simulink model "UNIFIER1"  (R2023b)
settings: Solver=ode1  StartTime=0.0  StopTime=t_sim  FixedStep=1/500  RelTol=1e-3
values from neighbouring files (symbols this model uses):
  b = 20.11467    [UNIFIERLanding_20240613_190735.mat]    (also in UNIFIER_LOAD.m; UNIFIER_LOADsim.m; UNIFIER_trim_out_20240612_032607.mat)
  c = 1.43676    [UNIFIERLanding_20240613_190735.mat]    (also in UNIFIER_LOAD.m; UNIFIER_LOADsim.m; UNIFIER_trim_out_20240612_032607.mat)
  DEP_INTEG_IC = 117.49388    [UNIFIER_LOAD.m]    (also in UNIFIER_LOADsim.m; UNIFIER_trim_out_20240612_032607.mat)
  dp_DEP =     [UNIFIERLanding_20240613_190735.mat]    (also in UNIFIER_trim_out_20240612_032607.mat)
  dp_FUSE_FIN =     [UNIFIER_trim_out_20240612_032607.mat]
  dp_HTU =     [UNIFIERLanding_20240613_190735.mat]    (also in UNIFIER_trim_out_20240612_032607.mat)
  dp_VTAIL =     [UNIFIER_trim_out_20240612_032607.mat]
  dp_VTAIL_INDUCED =     [UNIFIER_trim_out_20240612_032607.mat]
  dp_WING_root =     [UNIFIER_trim_out_20240612_032607.mat]
  dp_WING_tip =     [UNIFIER_trim_out_20240612_032607.mat]
  dumax = [1.0471975512 1.0471975512 1.0471975512 0.174532925199 2 2 2]    [UNIFIERLanding_20240613_190735.mat]
  Euler0 = xstar(7:9)'    [UNIFIER_6DOFsim_init.m]    (also in UNIFIER_LOAD.m = [0, 0, 0]; UNIFIER_LOADsim.m; UNIFIER_trim_out_20240612_032607.mat = [3.43106170069e-06 0.0515008506278 -2.79252663434])
  ground_alt = 0    [UNIFIER_LOAD.m]    (also in UNIFIER_LOADsim.m; UNIFIER_trim_out_20240612_032607.mat)
  m = 7057    [UNIFIERLanding_20240613_190735.mat]    (also in UNIFIER_LOAD.m; UNIFIER_LOADsim.m; UNIFIER_trim_out_20240612_032607.mat)
  omegab0 = xstar(10:12)'    [UNIFIER_6DOFsim_init.m]    (also in UNIFIER_LOAD.m = [0,0,0]; UNIFIER_LOADsim.m; UNIFIER_trim_out_20240612_032607.mat = [0 0 0])
  S = 29.98388    [UNIFIERLanding_20240613_190735.mat]    (also in UNIFIER_LOAD.m; UNIFIER_LOADsim.m; UNIFIER_trim_out_20240612_032607.mat)
  sensor_delay_steps = 5    [UNIFIER_LOAD.m]    (also in UNIFIER_LOADsim.m; UNIFIER_trim_out_20240612_032607.mat)
  solution =     [UNIFIERLanding_20240613_190735.mat]
  u1_0 = [ustar(1), -1*ustar(1), ustar(3)-ustar(2), ustar(3)+ustar(2), ustar(4), ustar(4)]    [UNIFIER_6DOFsim_init.m]    (also in UNIFIER_LOAD.m = [2.1112539e-05, -2.1112539e-05, -0.085004635, -0.084972650, ; UNIFIER_LOADsim.m = [2.1112539e-05, -2.1112539e-05, -0.085004635, -0.084972650, ; UNIFIER_trim_out_20240612_032607.mat = [2.1112539e-05 -2.1112539e-05 -0.085004635 -0.08497265 0.197)
  u2_0 = ones(1,12) .* ustar(5)    [UNIFIER_6DOFsim_init.m]    (also in UNIFIER_LOAD.m = ones(1,12) .* 0.4252; UNIFIER_LOADsim.m = ones(1,12) .* 0.4252; UNIFIER_trim_out_20240612_032607.mat = [0.4252 0.4252 0.4252 0.4252 0.4252 0.4252 0.4252 0.4252 0.4)
  u3_0 = ustar(7)    [UNIFIER_6DOFsim_init.m]    (also in UNIFIER_LOAD.m = 0.089689; UNIFIER_LOADsim.m = 0.089689; UNIFIER_trim_out_20240612_032607.mat = 0.089689)
  u4_0 = 0    [UNIFIER_6DOFsim_init.m]    (also in UNIFIER_LOAD.m; UNIFIER_LOADsim.m; UNIFIER_trim_out_20240612_032607.mat)
  u_trim = ustar    [UNIFIER_6DOFsim_init.m]    (also in UNIFIER_LOAD.m = [0.0; UNIFIER_LOADsim.m)
  umax = [0.436332312999 0.523598775598 0.523598775598 0.436332312999 1 1 1]    [UNIFIERLanding_20240613_190735.mat]    (also in UNIFIER_trim_out_20240612_032607.mat)
  umin = [-0.436332312999 -0.523598775598 -0.523598775598 0 0 -1 -0.5]    [UNIFIERLanding_20240613_190735.mat]    (also in UNIFIER_trim_out_20240612_032607.mat)
  Va = [72.7399985115 72.2978466179 70.3592089076 68.5755686022 67.5674222915 66.8967003826 65.8958642605 64.4243196248 62.667507398 61.0171213882 59.8601734245 59.2796795419 ... (250 elements, 250x1)]    [UNIFIERLanding_20240613_190735.mat]
  Vb0 = xstar(4:6)'    [UNIFIER_6DOFsim_init.m]    (also in UNIFIER_LOAD.m = [72.731047032614440, 0, 1.142307104518741]; UNIFIER_LOADsim.m; UNIFIER_trim_out_20240612_032607.mat = [52.6789583502 0 2.71559652634])
  vtail_dist_to_wing = 7.8070    (= 7.807)    [UNIFIER_LOAD.m]    (also in UNIFIER_LOADsim.m; UNIFIER_trim_out_20240612_032607.mat)
  vtail_nodes = [dp_VTAIL.Xs_LE;     dp_VTAIL.Ys_LE;     dp_VTAIL.Zs_LE]    [UNIFIER_LOAD.m]    (also in UNIFIER_LOADsim.m; UNIFIER_trim_out_20240612_032607.mat = [-16.4894695282 -2.83441376686 -2.73765826225 -16.1370849609)
  wing_nodes = [fliplr(dp_WING_tip.LE_Xs),fliplr(dp_WING_root.LE_Xs),dp_WING_root.LE_Xs,dp_WING_tip.LE_Xs;     fliplr(-dp_WING_tip.LE_Ys),fliplr(-dp_WING_root.LE_Ys),dp_WING_root.LE_Ys,dp_WING_tip.LE_Ys;     fliplr(dp_WING_tip.LE_Zs),fliplr(dp_WING_root.LE_Zs),dp_WING_root.LE_Zs,dp_WING_tip.LE_Zs]    [UNIFIER_LOAD.m]    (also in UNIFIER_LOADsim.m; UNIFIER_trim_out_20240612_032607.mat = [-7.70795631409 -9.67500019073 -0.98178178072 -7.66801691055)
  Xe0 = xstar(1:3)'    [UNIFIER_6DOFsim_init.m]    (also in UNIFIER_LOAD.m = [0,0,-1219]; UNIFIER_LOADsim.m; UNIFIER_trim_out_20240612_032607.mat = [0 0 -1100])
  xyz_cg = [-8.09 0 -0.2]    [UNIFIERLanding_20240613_190735.mat]    (also in UNIFIER_LOAD.m = [-8.09,0,-0.2]; UNIFIER_LOADsim.m = [-8.09,0,-0.2]; UNIFIER_trim_out_20240612_032607.mat)
  xyz_DEP = [-6.9629998 -10.05 -0.90899998 -6.921 -8.4499998 -0.792 -6.8660002 -6.8499999 -0.82300001 -6.8099999 -5.25 -0.85000002 ... (36 elements, 3x12)]    [UNIFIERLanding_20240613_190735.mat]    (also in UNIFIER_LOAD.m = [ -6.9629998	-6.9210000	-6.8660002	-6.8099999	-6.7540002	-6.; UNIFIER_LOADsim.m = [ -6.9629998	-6.9210000	-6.8660002	-6.8099999	-6.7540002	-6.; UNIFIER_trim_out_20240612_032607.mat)
undefined symbols (not defined in the file or in its folder): Earth, F, MIL, WGS84
libraries: simulink_extras x22, aerolibactuator x16, dspnetwork x15, sharedutil x14, sharedtransform x7, aerolibtransform2 x5, slpidlib x5, simulink x5, aerolibwind2 x4, matrix_library x1, shared6dof x1, aerolibatmos2 x1
(part 1 of 5)
settings Model: PauseTimes=1.5  Creator=johannes  LastModifiedBy=Reggie Johanes
settings DebuggingCC: ParameterPrecisionLossMsg=none  UnconnectedInputMsg=warning  UnconnectedOutputMsg=warning  UnconnectedLineMsg=warning  UnitsInconsistencyMsg=none  AllowAutomaticUnitConversions=off
settings ModelReferenceCC: EnableRefExpFcnMdlSchedulingChecks=on
settings RTWCC: DLArmComputeVersion=19.05

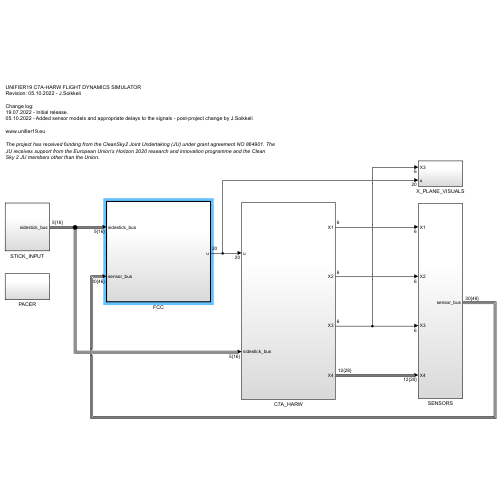
[thumbnail: Simulink's stored preview of the top-level diagram]
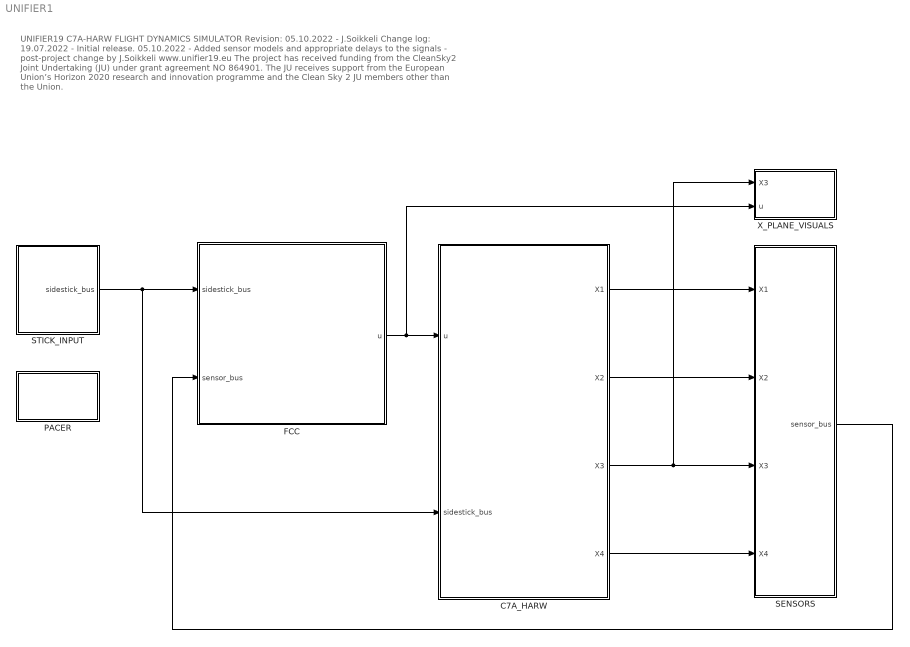
== system UNIFIER1 ==
  note: UNIFIER19 C7A-HARW FLIGHT DYNAMICS SIMULATOR
      | Revision: 05.10.2022 - J.Soikkeli
      |
      | Change log:
      | 19.07.2022 - Initial release.
      | 05.10.2022 - Added sensor models and appropriate delays to the signals - post-project change by J.Soikkeli
      |
      | www.unifier19.eu
      |
      | The project has received funding from the CleanSky2 Joint Undertaking (JU) under grant agreement NO 864901. The JU receives support from the European Union’s Horizon 2020 research and innovation programme and the Clean Sky 2 JU members other than the Union.
  C7A_HARW : Subsystem
  FCC : Subsystem  TreatAsAtomicUnit=on
  PACER : Subsystem
  SENSORS : Subsystem
  STICK_INPUT : Subsystem
  X_PLANE_VISUALS : Subsystem
  wires:
  C7A_HARW/3(X3) -> SENSORS/3(X3), X_PLANE_VISUALS/1(X3)
  FCC/1(u) -> X_PLANE_VISUALS/2(u), C7A_HARW/1(u)
  C7A_HARW/1(X1) -> SENSORS/1(X1)
  C7A_HARW/2(X2) -> SENSORS/2(X2)
  C7A_HARW/4(X4) -> SENSORS/4(X4)
  SENSORS/1(sensor_bus) -> FCC/2(sensor_bus)
  STICK_INPUT/1(sidestick_bus) -> C7A_HARW/2(sidestick_bus), FCC/1(sidestick_bus)

== system UNIFIER1/C7A_HARW ==
  u : Inport
  sidestick_bus : Inport  Port=2
  Actuator processing and transport delay 10 ms : Delay  DelayLength=5  InitialCondition=repmat([u1_0,u2_0,u3_0,u4_0]',1,5)
  Aero : Subsystem
  Bus Selector : BusSelector  OutputSignals=V_rw_tas,omega_rw,V_rw_mag_tas,beta,alpha,rho
  Cast{1,6..12} (8 alike) : DataTypeConversion  OutDataTypeStr=single  SaturateOnIntegerOverflow=off  RndMeth=Floor
  Demux : Demux  Outputs=[6,12,1,1]
  EOMandEnviroment1 : Subsystem
  FCC frame delay 10 ms (assumed 100Hz FCC) : Delay  DelayLength=5  InitialCondition=repmat([u1_0,u2_0,u3_0,u4_0]',1,5)
  Scopes : Subsystem
  Subsystems : Subsystem
  Sum : Sum  Inputs=|++
  Sum1 : Sum  Inputs=|++
  X1 : Outport
  X2 : Outport  Port=2
  X3 : Outport  Port=3
  X4 : Outport  Port=4
  wires:
  Aero/2(M) -> Sum1/1
  Bus Selector/1 -> Cast7/1  "<V_rw_tas>"
  Bus Selector/6 -> Cast8/1  "<rho>"
  Bus Selector/2 -> Cast9/1  "<omega_rw>"
  Cast6/1 -> Aero/7(DEP_J)
  Subsystems/1(DEP_J) -> Cast6/1
  Subsystems/3(F) -> Sum/2
  Aero/1(F) -> Sum/1
  Sum/1 -> EOMandEnviroment1/1(F)
  Sum1/1 -> EOMandEnviroment1/2(M)
  Subsystems/4(M) -> Sum1/2
  Bus Selector/3 -> Cast10/1  "<V_rw_mag_tas>"
  Bus Selector/4 -> Cast11/1  "<beta>"
  Bus Selector/5 -> Cast12/1  "<alpha>"
  Cast7/1 -> Aero/1(V_rw_tas)
  Cast8/1 -> Aero/6(rho)
  Cast9/1 -> Aero/2(omega_rw)
  Cast10/1 -> Aero/3(V_rw_mag_tas)
  Cast11/1 -> Aero/4(beta)
  Cast12/1 -> Aero/5(alpha)
  Cast1/1 -> Aero/8(u1 (rad))
  Subsystems/2(u1_out (rad)) -> Cast1/1
  EOMandEnviroment1/1(X1) -> Scopes/1(X1), X1/1
  EOMandEnviroment1/4(X4) -> Scopes/4(X4), X4/1, Subsystems/1(X4), Bus Selector/1
  EOMandEnviroment1/2(X2) -> Subsystems/7(X2), X2/1, Scopes/2(X2)
  EOMandEnviroment1/3(X3) -> Subsystems/6(X3), X3/1, Scopes/3(X3)
  Demux/4 -> Aero/9(u4 (gear))
  sidestick_bus/1 -> Subsystems/5(sidestick_bus)
  Demux/3 -> Subsystems/4(u3 (actf))
  Demux/2 -> Subsystems/3(u2 (actf))
  Demux/1 -> Subsystems/2(u1_in (rad))
  u/1 -> FCC frame delay 10 ms (assumed 100Hz FCC)/1
  FCC frame delay 10 ms (assumed 100Hz FCC)/1 -> Actuator processing and transport delay 10 ms/1
  Actuator processing and transport delay 10 ms/1 -> Demux/1

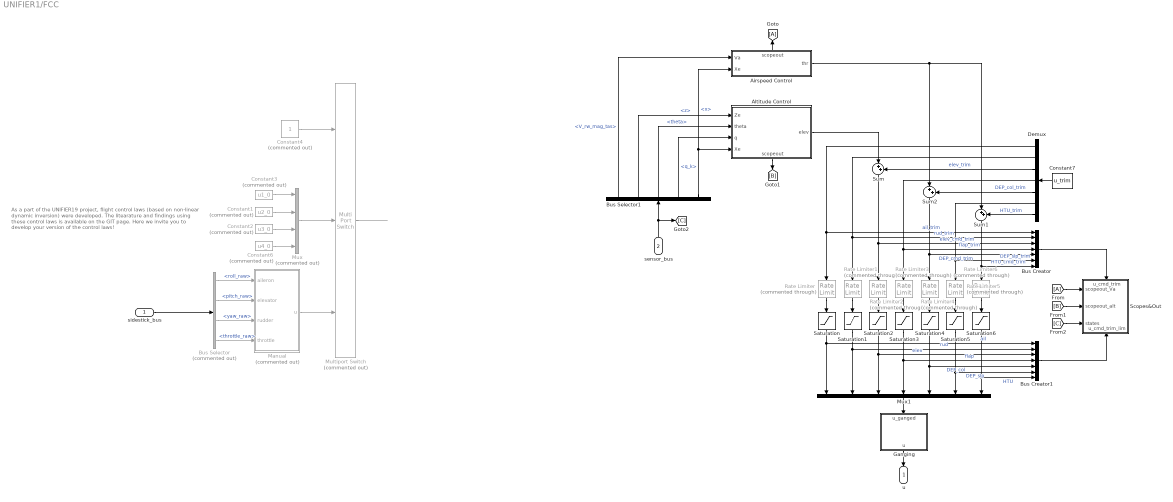
== system UNIFIER1/FCC ==
  note: As a part of the UNIFIER19 project, flight control laws (based on non-linear dynamic inversion) were developed. The litearature and findings using these control laws is available on the GIT page.
      |
      | Here we invite you to develop your version of the control laws!
  sidestick_bus : Inport
  sensor_bus : Inport  Port=2
  Airspeed Control : Subsystem
      settings: PortSchema="{\"entries\":[{\"content\":{\"sides\":[{\"content\":{\"connectorIds\":[\"In1\",\"In2\"]},\"type\":\"ConnectorPlacement.EquallySpacedRectSide\",\"uuid\":\"a3fb04a8-89c2-4134-89d4-6d6a43062b9b\"},{\"content\":{\"connectorIds\":[\"Out1\"],\"side\":\"RIGHT\"},\"type\":\"ConnectorPlacement.EquallySpacedRectSide\",\"uuid\":\"0d35a5ec-1bbb-45b5-ad25-2bc644cb46ec\"},{\"content\":{\"connectorIds\":[\"Out2\"],\"side\":\"TOP\"},\"type\":\"ConnectorPlacement.EquallySpacedRectSide\",\"uuid\":\"07800402-c5fd-46cf-bb6b-6507cb62190b\"}]},\"type\":\"ConnectorPlacement.EquallySpacedConnector\",\"uuid\":\"0f781fd0-6236-48b8-b612-1777b9bca292\"}],\"packageUris\":[\"http://schema.mathworks.com/mf0/Connector/R2020b\"],\"version\":\"1.0\"}"
  Altitude Control : Subsystem
      settings: PortSchema="{\"entries\":[{\"content\":{\"sides\":[{\"content\":{\"connectorIds\":[\"In1\",\"In2\",\"In3\",\"In4\"]},\"type\":\"ConnectorPlacement.EquallySpacedRectSide\",\"uuid\":\"d6eebd62-3574-4a6b-be51-6258a51c0c28\"},{\"content\":{\"connectorIds\":[\"Out1\"],\"side\":\"RIGHT\"},\"type\":\"ConnectorPlacement.EquallySpacedRectSide\",\"uuid\":\"54870a02-b95d-471b-a2c8-ee83b599c45e\"},{\"content\":{\"side\":\"TOP\"},\"type\":\"ConnectorPlacement.EquallySpacedRectSide\",\"uuid\":\"efdc830e-c8bf-412c-9d86-dbb1e6c1c86b\"},{\"content\":{\"connectorIds\":[\"Out2\"],\"side\":\"BOTTOM\"},\"type\":\"ConnectorPlacement.EquallySpacedRectSide\",\"uuid\":\"beb3ac17-a4c7-4320-a029-baa0478db22b\"}]},\"type\":\"ConnectorPlacement.EquallySpacedConnector\",\"uuid\":\"0f69f6a5-bc47-4551-ad8e-935190b4abb2\"}],\"packageUris\":[\"http://schema.mathworks.com/mf0/Connector/R2020b\"],\"version\":\"1.0\"}"
  Bus Creator : BusCreator  Inputs=7
  Bus Creator1 : BusCreator  Inputs=7
  Bus Selector : BusSelector  Commented=on  OutputSignals=roll_raw,pitch_raw,yaw_raw,throttle_raw
  Bus Selector1 : BusSelector  OutputSignals=V_rw_mag_tas,z,theta,q_k,x
  Constant1 : Constant  Commented=on  Value=u2_0
  Constant2 : Constant  Commented=on  Value=u3_0
  Constant3 : Constant  Commented=on  Value=u1_0
  Constant4 : Constant  Commented=on  SampleTime=-1
  Constant6 : Constant  Commented=on  Value=u4_0
  Constant7 : Constant  Value=u_trim
  Demux : Demux  Outputs=7
  From : From
  Ganging : Subsystem
  Goto : Goto
  Manual : Subsystem  Commented=on
  Multiport Switch : MultiPortSwitch  Commented=on  Inputs=2  SaturateOnIntegerOverflow=off  InputSameDT=off
  Mux : Mux  Commented=on
  Mux1 : Mux  Inputs=7
  Rate Limiter : RateLimiter  Commented=through  RisingSlewLimit=dumax(1)  FallingSlewLimit=-dumax(1)  SampleTimeMode=inherited
  Rate Limiter1 : RateLimiter  Commented=through  RisingSlewLimit=dumax(2)  FallingSlewLimit=-dumax(2)  SampleTimeMode=inherited
  Rate Limiter2 : RateLimiter  Commented=through  RisingSlewLimit=dumax(3)  FallingSlewLimit=-dumax(3)  SampleTimeMode=inherited
  Rate Limiter3 : RateLimiter  Commented=through  RisingSlewLimit=dumax(4)  FallingSlewLimit=-dumax(4)  SampleTimeMode=inherited
  Rate Limiter4 : RateLimiter  Commented=through  RisingSlewLimit=dumax(5)  FallingSlewLimit=-dumax(5)  SampleTimeMode=inherited
  Rate Limiter5 : RateLimiter  Commented=through  RisingSlewLimit=dumax(6)  FallingSlewLimit=-dumax(6)  SampleTimeMode=inherited
  Rate Limiter6 : RateLimiter  Commented=through  RisingSlewLimit=dumax(7)  FallingSlewLimit=-dumax(7)  SampleTimeMode=inherited
  Saturation : Saturate  UpperLimit=umax(1)  LowerLimit=umin(1)
  Saturation1 : Saturate  UpperLimit=umax(2)  LowerLimit=umin(2)
  Saturation2 : Saturate  UpperLimit=umax(3)  LowerLimit=umin(3)
  Saturation3 : Saturate  UpperLimit=umax(4)  LowerLimit=umin(4)
  Saturation4 : Saturate  UpperLimit=umax(5)  LowerLimit=umin(5)
  Saturation5 : Saturate  UpperLimit=umax(6)  LowerLimit=umin(6)
  Saturation6 : Saturate  UpperLimit=umax(7)  LowerLimit=umin(7)
  Scopes&Out : Subsystem
      settings: PortSchema="{\"entries\":[{\"content\":{\"sides\":[{\"content\":{\"connectorIds\":[\"In1\",\"In2\",\"In3\"]},\"type\":\"ConnectorPlacement.EquallySpacedRectSide\",\"uuid\":\"9c320b89-1cdf-46a8-9001-4899d9265a08\"},{\"content\":{\"side\":\"RIGHT\"},\"type\":\"ConnectorPlacement.EquallySpacedRectSide\",\"uuid\":\"9f59574f-7d1d-4902-b616-eb94195d59ee\"},{\"content\":{\"connectorIds\":[\"In4\"],\"side\":\"TOP\"},\"type\":\"ConnectorPlacement.EquallySpacedRectSide\",\"uuid\":\"0802dcde-7117-4a51-8755-c38da5aaf345\"},{\"content\":{\"connectorIds\":[\"In5\"],\"side\":\"BOTTOM\"},\"type\":\"ConnectorPlacement.EquallySpacedRectSide\",\"uuid\":\"322f023d-fcca-4329-b22d-247bcb46a2a3\"}]},\"type\":\"ConnectorPlacement.EquallySpacedConnector\",\"uuid\":\"183cf95f-4342-4e51-9921-cf7b583031df\"}],\"packageUris\":[\"http://schema.mathworks.com/mf0/Connector/R2020b\"],\"version\":\"1.0\"}"
  Sum : Sum  Inputs=|++
  Sum1 : Sum  Inputs=|++
  Sum2 : Sum  Inputs=|++
  u : Outport
  wires:
  Multiport Switch/1 -> ?
  Constant3/1 -> Mux/1
  Constant1/1 -> Mux/2
  Constant2/1 -> Mux/3
  Mux/1 -> Multiport Switch/2
  Bus Selector/1 -> Manual/1(aileron)  "<roll_raw>"
  Bus Selector/2 -> Manual/2(elevator)  "<pitch_raw>"
  Bus Selector/3 -> Manual/3(rudder)  "<yaw_raw>"
  Bus Selector/4 -> Manual/4(throttle)  "<throttle_raw>"
  Constant4/1 -> Multiport Switch/1
  Manual/1(u) -> Multiport Switch/3
  Constant6/1 -> Mux/4
  sidestick_bus/1 -> Bus Selector/1
  sensor_bus/1 -> Bus Selector1/1, [C]
  Ganging/1(u) -> u/1
  Bus Selector1/2 -> Altitude Control/1(Ze)  "<z>"
  Bus Selector1/3 -> Altitude Control/2(theta)  "<theta>"
  Bus Selector1/4 -> Altitude Control/3(q)  "<q_k>"
  Bus Selector1/1 -> Airspeed Control/1(Va)  "<V_rw_mag_tas>"
  Mux1/1 -> Ganging/1(u_ganged)
  Altitude Control/1(elev) -> Sum/1
  Airspeed Control/1(thr) -> Sum1/1, Sum2/1
  Saturation/1 -> Mux1/1, Bus Creator1/1  "ail"
  Saturation1/1 -> Mux1/2, Bus Creator1/2  "rud"
  Saturation2/1 -> Mux1/3, Bus Creator1/3  "elev"
  Saturation3/1 -> Mux1/4, Bus Creator1/4  "flap"
  Saturation4/1 -> Mux1/5, Bus Creator1/5  "DEP_col"
  Saturation5/1 -> Mux1/6, Bus Creator1/6  "DEP_slp"
  Saturation6/1 -> Mux1/7, Bus Creator1/7  "HTU"
  Constant7/1 -> Demux/1
  Demux/1 -> Bus Creator/1, Rate Limiter/1  "ail_trim"
  Demux/2 -> Bus Creator/2, Rate Limiter1/1  "rud_trim"
  Demux/3 -> Sum/2  "elev_trim"
  Demux/4 -> Bus Creator/4, Rate Limiter3/1  "flap_trim"
  Demux/5 -> Sum2/2  "DEP_col_trim"
  Demux/6 -> Bus Creator/6, Rate Limiter5/1  "DEP_slp_trim"
  Demux/7 -> Sum1/2  "HTU_trim"
  Bus Selector1/5 -> Altitude Control/4(Xe), Airspeed Control/2(Xe)  "<x>"
  Sum/1 -> Rate Limiter2/1, Bus Creator/3  "elev_cmd_trim"
  Sum1/1 -> Rate Limiter6/1, Bus Creator/7  "HTU_cmd_trim"
  Sum2/1 -> Rate Limiter4/1, Bus Creator/5  "DEP_cmd_trim"
  Rate Limiter/1 -> Saturation/1
  Rate Limiter1/1 -> Saturation1/1
  Rate Limiter2/1 -> Saturation2/1
  Rate Limiter3/1 -> Saturation3/1
  Rate Limiter4/1 -> Saturation4/1
  Rate Limiter5/1 -> Saturation5/1
  Rate Limiter6/1 -> Saturation6/1
  Altitude Control/2(scopeout) -> [B]
  Airspeed Control/2(scopeout) -> Goto/1
  From/1 -> Scopes&Out/1(scopeout_Va)
  [B] -> Scopes&Out/2(scopeout_alt)
  Bus Creator/1 -> Scopes&Out/4(u_cmd_trim)
  Bus Creator1/1 -> Scopes&Out/5(u_cmd_trim_lim)
  [C] -> Scopes&Out/3(states)

== system UNIFIER1/PACER ==
  note: Soft real time block and associated
      | s-function source codes:
      | - sfun_sleep.c
      | - sfun_getSystemClockTimeval.c
      | - sfun_output_to_console.c
      | are copyrighted
      | by Marc Compere
      | comperem@gmail.com
      | created : 28 May 2018
      | modified: 28 May 2018
  Constant1 : Constant  Value=0
  Constant2 : Constant
  Display : Display
  Manual Switch1 : ManualSwitch  CurrentSetting=0
  Mux : Mux  Inputs=3
  Output to Console : Subsystem  TreatAsAtomicUnit=on
  Subsystem : Subsystem
      settings: OpenFcn=h_fixed=0.001
      mask Display: fprintf('Double-Click to init\nstepsize variable, h_fixed')
  "pace error (s) " : Scope
  simulation time (s)1 : Clock
  soft real time subsystem : Subsystem  mask{t_sample=0.01}
      mask prompts: t_sample "Sleep function interval (s)"
  wires:
  soft real time subsystem/2(pace error (s)) -> "pace error (s) "/1, Display/1, Mux/3
  simulation time (s)1/1 -> Mux/1
  soft real time subsystem/1(t_elapsed_wall_clock (s)) -> Mux/2
  Constant1/1 -> Manual Switch1/2
  Mux/1 -> Output to Console/1(data to console)
  Constant2/1 -> Manual Switch1/1
  Manual Switch1/1 -> Output to Console/Enable

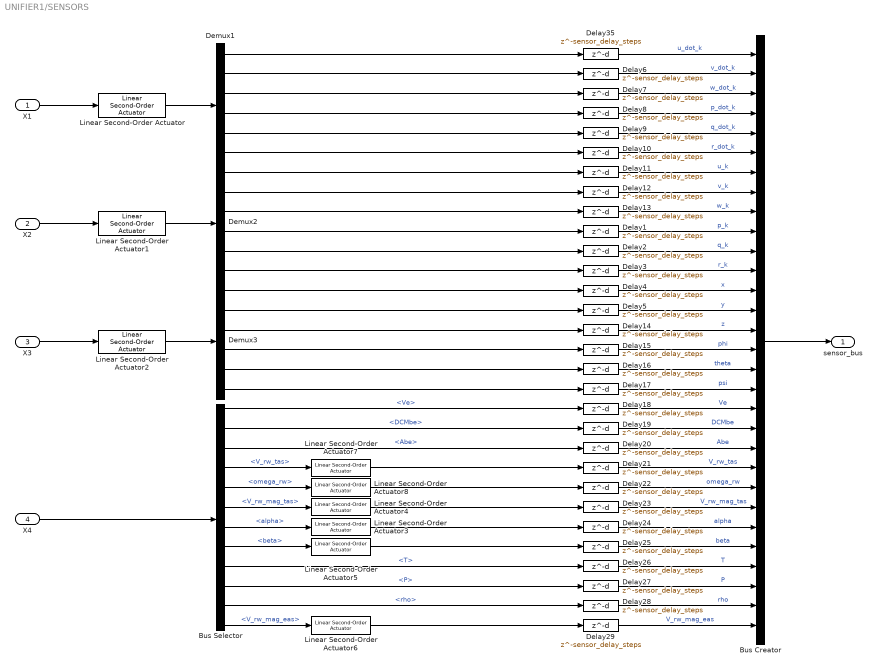
== system UNIFIER1/SENSORS ==
  X1 : Inport
  X2 : Inport  Port=2
  X3 : Inport  Port=3
  X4 : Inport  Port=4
  Bus Creator : BusCreator  Inputs=30
  Bus Selector : BusSelector  OutputSignals=Ve,DCMbe,Abe,V_rw_tas,omega_rw,V_rw_mag_tas,alpha,beta,T,P,rho,V_rw_mag_eas
  Delay{1..3,6..10,35} (9 alike) : Delay  DelayLength=sensor_delay_steps
  Delay11 : Delay  DelayLength=sensor_delay_steps  InitialCondition=Vb0(1)
  Delay12 : Delay  DelayLength=sensor_delay_steps  InitialCondition=Vb0(2)
  Delay13 : Delay  DelayLength=sensor_delay_steps  InitialCondition=Vb0(3)
  Delay14 : Delay  DelayLength=sensor_delay_steps  InitialCondition=Xe0(3)
  Delay15 : Delay  DelayLength=sensor_delay_steps  InitialCondition=Euler0(1)
  Delay16 : Delay  DelayLength=sensor_delay_steps  InitialCondition=Euler0(2)
  Delay17 : Delay  DelayLength=sensor_delay_steps  InitialCondition=Euler0(3)
  Delay18 : Delay  DelayLength=sensor_delay_steps  InitialCondition=repmat(Vb0',1,sensor_delay_steps)
  Delay19 : Delay  DelayLength=sensor_delay_steps  InitialCondition=0
  Delay20 : Delay  DelayLength=sensor_delay_steps  InitialCondition=0
  Delay21 : Delay  DelayLength=sensor_delay_steps  InitialCondition=repmat(Vb0',1,sensor_delay_steps)
  Delay22 : Delay  DelayLength=sensor_delay_steps  InitialCondition=0
  Delay23 : Delay  DelayLength=sensor_delay_steps  InitialCondition=sqrt(dot(Vb0,Vb0))
  Delay24 : Delay  DelayLength=sensor_delay_steps  InitialCondition=atan(Vb0(3)/Vb0(1))
  Delay25 : Delay  DelayLength=sensor_delay_steps  InitialCondition=asin(Vb0(2)/sqrt(dot(Vb0,Vb0)))
  Delay26 : Delay  DelayLength=sensor_delay_steps  InitialCondition=273
  Delay27 : Delay  DelayLength=sensor_delay_steps  InitialCondition=101325
  Delay28 : Delay  DelayLength=sensor_delay_steps  InitialCondition=1.225
  Delay29 : Delay  DelayLength=sensor_delay_steps  InitialCondition=sqrt(dot(Vb0,Vb0))
  Delay4 : Delay  DelayLength=sensor_delay_steps  InitialCondition=Xe0(1)
  Delay5 : Delay  DelayLength=sensor_delay_steps  InitialCondition=Xe0(2)
  Demux1 : Demux  Outputs=6
  Demux2 : Demux  Outputs=6
  Demux3 : Demux  Outputs=6
  Linear Second-Order Actuator : aerolibactuator/Linear Second-Order Actuator  wn_fin=30*2*pi  z_fin=1  fin_act_0=zeros(1,6)  fin_act_vel=0
  Linear Second-Order Actuator1 : aerolibactuator/Linear Second-Order Actuator  wn_fin=30*2*pi  z_fin=1  fin_act_0=[Vb0,omegab0]  fin_act_vel=0
  Linear Second-Order Actuator2 : aerolibactuator/Linear Second-Order Actuator  wn_fin=30*2*pi  z_fin=1  fin_act_0=[Xe0,Euler0]  fin_act_vel=0
  Linear Second-Order Actuator3 : aerolibactuator/Linear Second-Order Actuator  wn_fin=5*2*pi  z_fin=1  fin_act_0=atan(Vb0(3)/Vb0(1))  fin_act_vel=0
  Linear Second-Order Actuator4 : aerolibactuator/Linear Second-Order Actuator  wn_fin=5*2*pi  z_fin=1  fin_act_0=sqrt((Vb0(1)^2+Vb0(2)^2+Vb0(3)^2))  fin_act_vel=0
  Linear Second-Order Actuator5 : aerolibactuator/Linear Second-Order Actuator  wn_fin=5*2*pi  z_fin=1  fin_act_0=asin(Vb0(2)/sqrt((Vb0(1)^2+Vb0(2)^2+Vb0(3)^2)))  fin_act_vel=0
  Linear Second-Order Actuator6 : aerolibactuator/Linear Second-Order Actuator  wn_fin=5*2*pi  z_fin=1  fin_act_0=sqrt((Vb0(1)^2+Vb0(2)^2+Vb0(3)^2))  fin_act_vel=0
  Linear Second-Order Actuator7 : aerolibactuator/Linear Second-Order Actuator  wn_fin=5*2*pi  z_fin=1  fin_act_0=Vb0  fin_act_vel=0
  Linear Second-Order Actuator8 : aerolibactuator/Linear Second-Order Actuator  wn_fin=30*2*pi  z_fin=1  fin_act_0=omegab0  fin_act_vel=0
  sensor_bus : Outport
  wires:
  Demux1/1 -> Delay35/1
  Demux1/2 -> Delay6/1
  X4/1 -> Bus Selector/1
  Bus Selector/4 -> Linear Second-Order Actuator7/1  "<V_rw_tas>"
  Bus Selector/5 -> Linear Second-Order Actuator8/1  "<omega_rw>"
  Bus Selector/6 -> Linear Second-Order Actuator4/1  "<V_rw_mag_tas>"
  Bus Selector/7 -> Linear Second-Order Actuator3/1  "<alpha>"
  Bus Selector/8 -> Linear Second-Order Actuator5/1  "<beta>"
  Bus Selector/12 -> Linear Second-Order Actuator6/1  "<V_rw_mag_eas>"
  X1/1 -> Linear Second-Order Actuator/1
  X2/1 -> Linear Second-Order Actuator1/1
  X3/1 -> Linear Second-Order Actuator2/1
  Linear Second-Order Actuator/1 -> Demux1/1
  Linear Second-Order Actuator1/1 -> Demux2/1
  Linear Second-Order Actuator2/1 -> Demux3/1
  Bus Creator/1 -> sensor_bus/1
  Linear Second-Order Actuator6/1 -> Delay29/1
  Bus Selector/11 -> Delay28/1  "<rho>"
  Bus Selector/10 -> Delay27/1  "<P>"
  Bus Selector/9 -> Delay26/1  "<T>"
  Linear Second-Order Actuator5/1 -> Delay25/1
  Linear Second-Order Actuator3/1 -> Delay24/1
  Linear Second-Order Actuator4/1 -> Delay23/1
  Linear Second-Order Actuator8/1 -> Delay22/1
  Linear Second-Order Actuator7/1 -> Delay21/1
  Bus Selector/3 -> Delay20/1  "<Abe>"
  Bus Selector/2 -> Delay19/1  "<DCMbe>"
  Bus Selector/1 -> Delay18/1  "<Ve>"
  Demux3/6 -> Delay17/1
  Demux3/5 -> Delay16/1
  Demux3/4 -> Delay15/1
  Demux3/3 -> Delay14/1
  Demux3/2 -> Delay5/1
  Demux3/1 -> Delay4/1
  Demux2/6 -> Delay3/1
  Demux2/5 -> Delay2/1
  Demux2/4 -> Delay1/1
  Demux2/3 -> Delay13/1
  Demux2/2 -> Delay12/1
  Demux2/1 -> Delay11/1
  Demux1/6 -> Delay10/1
  Demux1/5 -> Delay9/1
  Demux1/4 -> Delay8/1
  Demux1/3 -> Delay7/1
  Delay35/1 -> Bus Creator/1  "u_dot_k"
  Delay6/1 -> Bus Creator/2  "v_dot_k"
  Delay7/1 -> Bus Creator/3  "w_dot_k"
  Delay8/1 -> Bus Creator/4  "p_dot_k"
  Delay9/1 -> Bus Creator/5  "q_dot_k"
  Delay10/1 -> Bus Creator/6  "r_dot_k"
  Delay11/1 -> Bus Creator/7  "u_k"
  Delay12/1 -> Bus Creator/8  "v_k"
  Delay13/1 -> Bus Creator/9  "w_k"
  Delay1/1 -> Bus Creator/10  "p_k"
  Delay2/1 -> Bus Creator/11  "q_k"
  Delay3/1 -> Bus Creator/12  "r_k"
  Delay4/1 -> Bus Creator/13  "x"
  Delay5/1 -> Bus Creator/14  "y"
  Delay14/1 -> Bus Creator/15  "z"
  Delay15/1 -> Bus Creator/16  "phi"
  Delay16/1 -> Bus Creator/17  "theta"
  Delay17/1 -> Bus Creator/18  "psi"
  Delay18/1 -> Bus Creator/19  "Ve"
  Delay19/1 -> Bus Creator/20  "DCMbe"
  Delay20/1 -> Bus Creator/21  "Abe"
  Delay21/1 -> Bus Creator/22  "V_rw_tas"
  Delay22/1 -> Bus Creator/23  "omega_rw"
  Delay23/1 -> Bus Creator/24  "V_rw_mag_tas"
  Delay24/1 -> Bus Creator/25  "alpha"
  Delay25/1 -> Bus Creator/26  "beta"
  Delay26/1 -> Bus Creator/27  "T"
  Delay27/1 -> Bus Creator/28  "P"
  Delay28/1 -> Bus Creator/29  "rho"
  Delay29/1 -> Bus Creator/30  "V_rw_mag_eas"

== system UNIFIER1/STICK_INPUT ==
  1-D Lookup Table : Lookup_n-D  NumberOfTableDimensions=1  BreakpointsForDimension1=[0,32770,65540]  IndexSearchMethod=Linear search  BeginIndexSearchUsingPreviousIndexResult=on  Table=[-1,0,1]  ExtrapMethod=Clip  RemoveProtectionInput=on  UseLastTableValue=on  InternalRulePriority=Speed  RndMeth=Simplest
  Bus Creator : BusCreator  Inputs=5
  Constant : Constant  Value=0.5
  Demux : Demux  Outputs=16
  Demux1 : Demux
  Gain : Gain  Gain=0.5
  Mux : Mux  Inputs=12
  Mux1 : Mux
  S-Function : S-Function  FunctionName=sfun_joyinfoex  SFunctionDeploymentMode=off  EnableBusSupport=off
  Sum : Sum  Inputs=++|
  Unary Minus : UnaryMinus
  deviceID : Constant  Value=0
  sidestick_bus : Outport
  wires:
  Demux1/2 -> Bus Creator/2  "pitch_raw"
  Demux1/1 -> Bus Creator/1  "roll_raw"
  Sum/1 -> Bus Creator/3  "throttle_raw"
  Bus Creator/1 -> sidestick_bus/1
  Demux1/4 -> Bus Creator/4  "yaw_raw"
  deviceID/1 -> S-Function/1
  S-Function/1 -> Demux/1
  Demux/5 -> Mux/1
  Demux/6 -> Mux/2
  Demux/7 -> Mux/3
  Demux/8 -> Mux/4
  Demux/9 -> Mux/5
  Demux/10 -> Mux/6
  Demux/11 -> Mux/7
  Demux/12 -> Mux/8
  Demux/13 -> Mux/9
  Demux/14 -> Mux/10
  Demux/15 -> Mux/11
  Demux/16 -> Mux/12
  Mux/1 -> Bus Creator/5  "buttons"
  Demux/1 -> Mux1/1
  Demux/2 -> Mux1/2
  Demux/3 -> Mux1/3
  Demux/4 -> Mux1/4
  Mux1/1 -> 1-D Lookup Table/1
  1-D Lookup Table/1 -> Demux1/1
  Gain/1 -> Sum/2
  Demux1/3 -> Unary Minus/1
  Unary Minus/1 -> Gain/1
  Constant/1 -> Sum/1

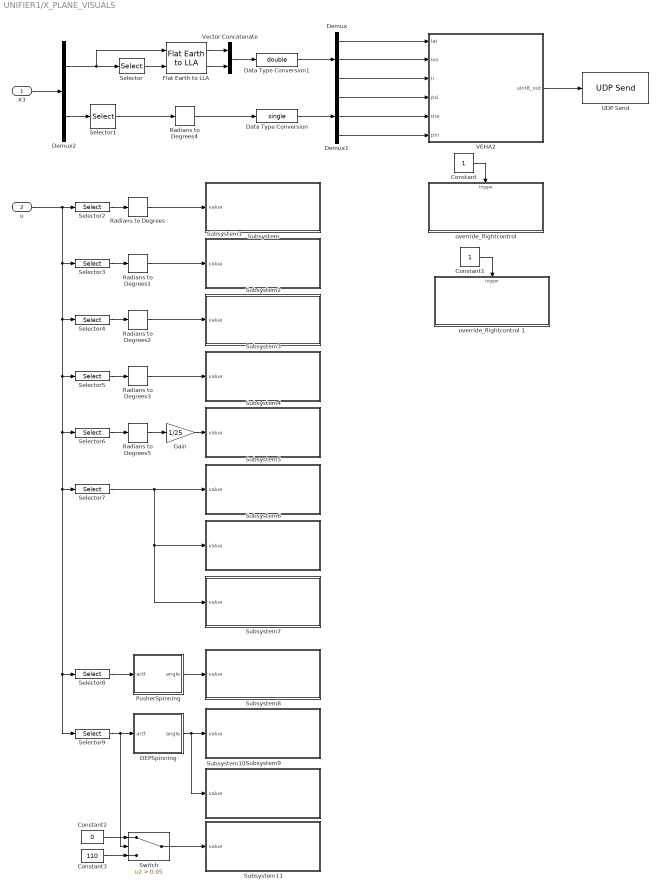
== system UNIFIER1/X_PLANE_VISUALS ==
  X3 : Inport
  u : Inport  Port=2
  Constant : Constant
  Constant1 : Constant
  Constant2 : Constant  Value=0
  Constant3 : Constant  Value=110
  DEPSpinning : Subsystem
  Data Type Conversion : DataTypeConversion  OutDataTypeStr=single  SaturateOnIntegerOverflow=off  RndMeth=Floor
  Data Type Conversion1 : DataTypeConversion  OutDataTypeStr=double  SaturateOnIntegerOverflow=off  RndMeth=Floor
  Demux : Demux  Outputs=3
  Demux1 : Demux  Outputs=3
  Demux2 : Demux  Outputs=2
  Flat Earth to LLA : aerolibtransform2/Flat Earth to LLA  units=Metric (MKS)  ptype=Earth (WGS84)  F=1/298.257223563  R=6378137  refPosPort=off  LL0=latlong0  psi=0
  Gain : Gain  Gain=1/25
  PusherSpinning : Subsystem
  Radians to Degrees{,1..5} (6 alike) : simulink_extras/Transformations/Radians to Degrees
  Selector : Selector  InputPortWidth=3  IndexOptions=Index vector (dialog)  Indices=[3]  OutputSizes=1
  Selector1 : Selector  InputPortWidth=3  IndexOptions=Index vector (dialog)  Indices=[3,2,1]  OutputSizes=1
  Selector2 : Selector  InputPortWidth=20  IndexOptions=Index vector (dialog)  Indices=1  OutputSizes=1
  Selector3 : Selector  InputPortWidth=20  IndexOptions=Index vector (dialog)  Indices=2  OutputSizes=1
  Selector4 : Selector  InputPortWidth=20  IndexOptions=Index vector (dialog)  Indices=3  OutputSizes=1
  Selector5 : Selector  InputPortWidth=20  IndexOptions=Index vector (dialog)  Indices=4  OutputSizes=1
  Selector6 : Selector  InputPortWidth=20  IndexOptions=Index vector (dialog)  Indices=5  OutputSizes=1
  Selector7 : Selector  InputPortWidth=20  IndexOptions=Index vector (dialog)  Indices=20  OutputSizes=1
  Selector8 : Selector  InputPortWidth=20  IndexOptions=Index vector (dialog)  Indices=19  OutputSizes=1
  Selector9 : Selector  InputPortWidth=20  IndexOptions=Index vector (dialog)  Indices=12  OutputSizes=1
  Subsystem : Subsystem  mask{str='sim/flightmodel/controls/wing1l_ail1def'}
      mask prompts: str "dref"
  Subsystem1 : Subsystem  mask{str='sim/flightmodel/controls/wing1r_ail1def'}
      mask prompts: str "dref"
  Subsystem10 : Subsystem  mask{str='AFormX/Unifier/DEP/PropAngDeg'}
      mask prompts: str "dref"
  Subsystem11 : Subsystem  mask{str='AFormX/Unifier/DEP/DEPAngle'}
      mask prompts: str "dref"
  Subsystem2 : Subsystem  mask{str='sim/flightmodel/controls/mwing02_elv1def'}
      mask prompts: str "dref"
  Subsystem3 : Subsystem  mask{str='sim/flightmodel/controls/mwing01_elv1def'}
      mask prompts: str "dref"
  Subsystem4 : Subsystem  mask{str='sim/flightmodel/controls/flaprat'}
      mask prompts: str "dref"
  Subsystem5 : Subsystem  mask{str='sim/aircraft/parts/acf_gear_deploy[0]'}
      mask prompts: str "dref"
  Subsystem6 : Subsystem  mask{str='sim/aircraft/parts/acf_gear_deploy[1]'}
      mask prompts: str "dref"
  Subsystem7 : Subsystem  mask{str='sim/aircraft/parts/acf_gear_deploy[2]'}
      mask prompts: str "dref"
  Subsystem8 : Subsystem  mask{str='sim/flightmodel2/engines/prop_rotation_angle_deg[0]'}
      mask prompts: str "dref"
  Subsystem9 : Subsystem  mask{str='sim/flightmodel2/engines/prop_rotation_angle_deg[1]'}
      mask prompts: str "dref"
  Switch : Switch  Criteria=u2 > Threshold  Threshold=0.05  SaturateOnIntegerOverflow=off  InputSameDT=off
  UDP Send : dspnetwork/UDP Send  remoteURL='127.0.0.1'  remotePort=49000  localURL='0.0.0.0'  localPortSource=Automatically determine  localPort=-1  sendBufferSize=8192  sampletime=-1  blockPlatform=[]  separateLengthPort=0
  VEHA2 : MATLAB Function  TreatAsAtomicUnit=on
  Vector Concatenate : Concatenate
  "override_flightcontrol " : Subsystem  TreatAsAtomicUnit=on
  override_flightcontrol 1 : Subsystem  TreatAsAtomicUnit=on
  wires:
  Demux/1 -> VEHA2/1(lat)
  Demux/2 -> VEHA2/2(lon)
  Data Type Conversion/1 -> Demux1/1
  Demux1/3 -> VEHA2/6(phi)
  Flat Earth to LLA/1 -> Vector Concatenate/1
  Selector/1 -> Flat Earth to LLA/2
  VEHA2/1(uint8_out) -> UDP Send/1
  Demux2/2 -> Selector1/1
  Demux1/1 -> VEHA2/4(psi)
  Demux1/2 -> VEHA2/5(the)
  Demux/3 -> VEHA2/3(h)
  Data Type Conversion1/1 -> Demux/1
  Vector Concatenate/1 -> Data Type Conversion1/1
  Flat Earth to LLA/2 -> Vector Concatenate/2
  Demux2/1 -> Selector/1, Flat Earth to LLA/1
  Radians to Degrees4/1 -> Data Type Conversion/1
  Selector1/1 -> Radians to Degrees4/1
  Constant/1 -> "override_flightcontrol "/Trigger
  X3/1 -> Demux2/1
  Selector2/1 -> Radians to Degrees/1
  Radians to Degrees/1 -> Subsystem/1(value)
  Selector3/1 -> Radians to Degrees1/1
  Radians to Degrees1/1 -> Subsystem1/1(value)
  u/1 -> Selector6/1, Selector9/1, Selector8/1, Selector7/1, Selector5/1, Selector4/1, Selector3/1, Selector2/1
  Constant1/1 -> override_flightcontrol 1/Trigger
  Selector4/1 -> Radians to Degrees2/1
  Radians to Degrees2/1 -> Subsystem2/1(value)
  Radians to Degrees3/1 -> Subsystem3/1(value)
  Selector5/1 -> Radians to Degrees3/1
  Radians to Degrees5/1 -> Gain/1
  Gain/1 -> Subsystem4/1(value)
  Selector6/1 -> Radians to Degrees5/1
  Selector7/1 -> Subsystem7/1(value), Subsystem6/1(value), Subsystem5/1(value)
  Selector8/1 -> PusherSpinning/1(actf)
  PusherSpinning/1(angle) -> Subsystem8/1(value)
  DEPSpinning/1(angle) -> Subsystem10/1(value), Subsystem9/1(value)
  Selector9/1 -> Switch/2, DEPSpinning/1(actf)
  Switch/1 -> Subsystem11/1(value)
  Constant2/1 -> Switch/1
  Constant3/1 -> Switch/3

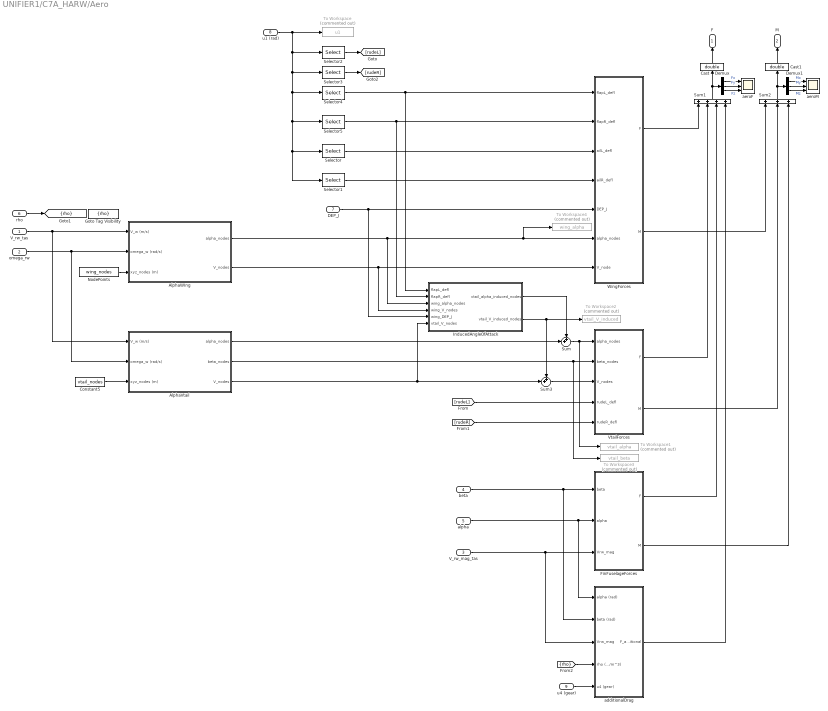
== system UNIFIER1/C7A_HARW/Aero ==
  V_rw_tas : Inport  OutDataTypeStr=single  Unit=m/s  PortDimensions=3  LockScale=on
  omega_rw : Inport  Port=2  OutDataTypeStr=single  Unit=rad/s  PortDimensions=3  LockScale=on
  V_rw_mag_tas : Inport  Port=3  OutDataTypeStr=single
  beta : Inport  Port=4  OutDataTypeStr=single
  alpha : Inport  Port=5  OutDataTypeStr=single
  rho : Inport  Port=6  OutDataTypeStr=single  Unit=kg/m^3  PortDimensions=1  LockScale=on
  DEP_J : Inport  Port=7  OutDataTypeStr=single  LockScale=on
  u1 (rad) : Inport  Port=8
  u4 (gear) : Inport  Port=9
  AlphaVtail : Subsystem  TreatAsAtomicUnit=on
  AlphaWIng : Subsystem  TreatAsAtomicUnit=on
  Cast : DataTypeConversion  OutDataTypeStr=double  SaturateOnIntegerOverflow=off  RndMeth=Floor
  Cast1 : DataTypeConversion  OutDataTypeStr=double  SaturateOnIntegerOverflow=off  RndMeth=Floor
  Constant5 : Constant  Value=vtail_nodes
  Demux : Demux  Outputs=3
  Demux1 : Demux  Outputs=3
  FinFuselageForces : Subsystem
  Goto Tag Visibility : GotoTagVisibility  GotoTag=rho
  InducedAngleOfAttack : Subsystem
  NodePoints : Constant  Value=wing_nodes
  Selector : Selector  InputPortWidth=6  IndexOptions=Index vector (dialog)  Indices=1  OutputSizes=1
  Selector1 : Selector  InputPortWidth=6  IndexOptions=Index vector (dialog)  Indices=2  OutputSizes=1
  Selector2 : Selector  InputPortWidth=6  IndexOptions=Index vector (dialog)  Indices=3  OutputSizes=1
  Selector3 : Selector  InputPortWidth=6  IndexOptions=Index vector (dialog)  Indices=4  OutputSizes=1
  Selector4 : Selector  InputPortWidth=6  IndexOptions=Index vector (dialog)  Indices=5  OutputSizes=1
  Selector5 : Selector  InputPortWidth=6  IndexOptions=Index vector (dialog)  Indices=6  OutputSizes=1
  Sum : Sum  Inputs=++|
  Sum1 : Sum  Inputs=++++
  Sum2 : Sum  Inputs=+++
  Sum3 : Sum  Inputs=++|
  To Workspace : ToWorkspace  Commented=on  VariableName=u1  SaveFormat=Structure With Time  SampleTime=1/100
  To Workspace1 : ToWorkspace  Commented=on  VariableName=vtail_alpha  SaveFormat=Structure With Time  SampleTime=1/100
  To Workspace2 : ToWorkspace  Commented=on  VariableName=vtail_V_induced  SaveFormat=Structure With Time  SampleTime=1/100
  To Workspace3 : ToWorkspace  Commented=on  VariableName=vtail_beta  SaveFormat=Structure With Time  SampleTime=1/100
  To Workspace4 : ToWorkspace  Commented=on  VariableName=wing_alpha  SaveFormat=Structure With Time  SampleTime=1/100
  VtailForces : Subsystem
  WingForces : Subsystem
  additionalDrag : Subsystem
  aeroF : Scope  NumInputPorts=3
  aeroM : Scope  NumInputPorts=3
  F : Outport  Unit=N  PortDimensions=3  LockScale=on
  M : Outport  Port=2  Unit=N*m  PortDimensions=3  LockScale=on
  tag scope: rho=scoped
  wires:
  NodePoints/1 -> AlphaWIng/3(xyz_nodes (m))
  Constant5/1 -> AlphaVtail/3(xyz_nodes (m))
  V_rw_tas/1 -> AlphaVtail/1(V_w (m/s)), AlphaWIng/1(V_w (m/s))
  omega_rw/1 -> AlphaVtail/2(omega_w (rad/s)), AlphaWIng/2(omega_w (rad/s))
  AlphaWIng/2(V_nodes) -> WingForces/7(V_node), InducedAngleOfAttack/4(wing_V_nodes)
  DEP_J/1 -> WingForces/5(DEP_J), InducedAngleOfAttack/5(wing_DEP_J)
  Sum/1 -> VtailForces/1(alpha_nodes), To Workspace1/1
  rho/1 -> [rho]
  AlphaVtail/2(beta_nodes) -> VtailForces/2(beta_nodes), To Workspace3/1
  [rudeL] -> VtailForces/4(rudeL_defl)
  [rudeR] -> VtailForces/5(rudeR_defl)
  WingForces/1(F) -> Sum1/1
  VtailForces/1(F) -> Sum1/2
  WingForces/2(M) -> Sum2/1
  VtailForces/2(M) -> Sum2/2
  Sum1/1 -> Demux/1, Cast/1
  AlphaVtail/3(V_nodes) -> InducedAngleOfAttack/6(vtail_V_nodes), Sum3/2
  InducedAngleOfAttack/1(vtail_alpha_induced_nodes) -> Sum/1
  InducedAngleOfAttack/2(vtail_V_induced_nodes) -> To Workspace2/1, Sum3/1
  Sum3/1 -> VtailForces/3(V_nodes)
  AlphaVtail/1(alpha_nodes) -> Sum/2
  Cast/1 -> F/1
  Cast1/1 -> M/1
  V_rw_mag_tas/1 -> FinFuselageForces/3(Vrw_mag), additionalDrag/3(Vrw_mag)
  beta/1 -> FinFuselageForces/1(beta), additionalDrag/2(beta (rad))
  FinFuselageForces/1(F) -> Sum1/3
  FinFuselageForces/2(M) -> Sum2/3
  Selector/1 -> WingForces/3(ailL_defl)
  Selector1/1 -> WingForces/4(ailR_defl)
  Selector4/1 -> WingForces/1(flapL_defl), InducedAngleOfAttack/1(flapL_defl)
  Selector5/1 -> WingForces/2(flapR_defl), InducedAngleOfAttack/2(flapR_defl)
  Selector2/1 -> [rudeL]
  Selector3/1 -> [rudeR]
  Demux/1 -> aeroF/1  "Fx"
  Demux/2 -> aeroF/2  "Fy"
  Demux/3 -> aeroF/3  "Fz"
  Sum2/1 -> Cast1/1, Demux1/1
  Demux1/2 -> aeroM/2  "My"
  Demux1/1 -> aeroM/1  "Mx"
  Demux1/3 -> aeroM/3  "Mz"
  AlphaWIng/1(alpha_nodes) -> WingForces/6(alpha_nodes), To Workspace4/1, InducedAngleOfAttack/3(wing_alpha_nodes)
  alpha/1 -> FinFuselageForces/2(alpha), additionalDrag/1(alpha (rad))
  [rho] -> additionalDrag/4(rho (kg/m^3))
  additionalDrag/1(F_additional) -> Sum1/4
  u4 (gear)/1 -> additionalDrag/5(u4 (gear))
  u1 (rad)/1 -> Selector1/1, Selector/1, Selector5/1, Selector4/1, Selector3/1, Selector2/1, To Workspace/1

== system UNIFIER1/C7A_HARW/EOMandEnviroment1 ==
  F : Inport
  M : Inport  Port=2
  Bus Creator : BusCreator  Inputs=12
  Conversion : Subsystem
  EOM: 6DOF (Euler Angles) : shared6dof/6DOF (Euler Angles)  units=Metric (MKS)  mtype=Fixed  rep=Euler Angles  xme_0=Xe0  Vm_0=Vb0  eul_0=Euler0  pm_0=omegab0  mass_0=m  mass_e=0.5  mass_f=2.0  inertia=I  inertia_e=eye(3)  inertia_f=2*eye(3)  k_quat=1.0  vre_flag=on  abi_flag=on  aMode=aMode  xme_statename=''  Vm_statename=''  eul_statename=''  quat_statename=''  pm_statename=''  mass_statename=''
  Enviroment : Subsystem
  Mux : Mux  Inputs=2
  Mux1 : Mux  Inputs=2
  Mux2 : Mux  Inputs=2
  To Workspace : ToWorkspace  Commented=on  VariableName=alpha  SaveFormat=Structure With Time  SampleTime=1/100
  To Workspace1 : ToWorkspace  Commented=on  VariableName=X3  SaveFormat=Structure With Time  SampleTime=1/100
  To Workspace2 : ToWorkspace  Commented=on  VariableName=X2  SaveFormat=Structure With Time  SampleTime=1/100
  To Workspace3 : ToWorkspace  Commented=on  VariableName=X1  SaveFormat=Structure With Time  SampleTime=1/100
  To Workspace4 : ToWorkspace  Commented=on  VariableName=beta  SaveFormat=Structure With Time  SampleTime=1/100
  To Workspace5 : ToWorkspace  Commented=on  VariableName=Vrw_mag  SaveFormat=Structure With Time  SampleTime=1/100
  X1 : Outport
  X2 : Outport  Port=2
  X3 : Outport  Port=3
  X4 : Outport  Port=4
  wires:
  EOM: 6DOF (Euler Angles)/5 -> Enviroment/2(Vb), Mux1/1  "Vb"
  EOM: 6DOF (Euler Angles)/3 -> Mux2/2  "Euler"
  Conversion/3(alpha) -> Bus Creator/7, To Workspace/1  "alpha"
  Mux2/1 -> To Workspace1/1, X3/1
  Enviroment/1(Vrw) -> Bus Creator/4, Conversion/1(Vrw)  "V_rw_tas"
  EOM: 6DOF (Euler Angles)/2 -> Enviroment/1(Xe), Mux2/1  "Xe"
  Enviroment/3(T) -> Bus Creator/9  "T"
  EOM: 6DOF (Euler Angles)/8 -> Mux/1  "Abb"
  Bus Creator/1 -> X4/1
  EOM: 6DOF (Euler Angles)/4 -> Enviroment/3(DCM), Bus Creator/2  "DCMbe"
  EOM: 6DOF (Euler Angles)/6 -> Enviroment/4(omega), Mux1/2  "omegadt"
  Conversion/4(beta) -> To Workspace4/1, Bus Creator/8  "beta"
  Enviroment/5(rho) -> Conversion/2(rho), Bus Creator/11  "rho"
  Conversion/1(Vrw_mag) -> To Workspace5/1, Bus Creator/6  "V_rw_mag_tas"
  EOM: 6DOF (Euler Angles)/7 -> Mux/2  "domegadtdt"
  EOM: 6DOF (Euler Angles)/9 -> Bus Creator/3  "Abe"
  Enviroment/2(omegaw) -> Bus Creator/5  "omega_rw"
  EOM: 6DOF (Euler Angles)/1 -> Bus Creator/1  "Ve"
  Enviroment/4(P) -> Bus Creator/10  "P"
  Mux1/1 -> X2/1, To Workspace2/1
  Mux/1 -> To Workspace3/1, X1/1
  Conversion/2(Vrw_mag_eas) -> Bus Creator/12  "V_rw_mag_eas"
  F/1 -> EOM: 6DOF (Euler Angles)/1
  M/1 -> EOM: 6DOF (Euler Angles)/2

== system UNIFIER1/C7A_HARW/Scopes ==
  X1 : Inport
  X2 : Inport  Port=2
  X3 : Inport  Port=3
  X4 : Inport  Port=4
  Bus Selector : BusSelector  OutputSignals=V_rw_mag_tas,V_rw_mag_eas,alpha,beta
  Demux : Demux  Outputs=6
  Demux1 : Demux  Outputs=6
  Demux2 : Demux  Outputs=6
  Radians to Degrees{,1..4} (5 alike) : simulink_extras/Transformations/Radians to Degrees
  Vrw_mag : Scope  NumInputPorts=2
  alphabeta : Scope  NumInputPorts=2
  phithetapsi : Scope  NumInputPorts=3
  pqr : Scope  NumInputPorts=3
  pqr_dot : Scope  NumInputPorts=3
  uvw : Scope  NumInputPorts=3
  uvw_dot : Scope  NumInputPorts=3
  xyz : Scope  NumInputPorts=3
  wires:
  X4/1 -> Bus Selector/1
  Bus Selector/3 -> Radians to Degrees/1  "<alpha>"
  Bus Selector/4 -> Radians to Degrees1/1  "<beta>"
  Bus Selector/1 -> Vrw_mag/1  "<V_rw_mag_tas>"
  Radians to Degrees/1 -> alphabeta/1
  Radians to Degrees1/1 -> alphabeta/2
  X1/1 -> Demux/1
  X2/1 -> Demux1/1
  X3/1 -> Demux2/1
  Demux/1 -> uvw_dot/1
  Demux/2 -> uvw_dot/2
  Demux/3 -> uvw_dot/3
  Demux/4 -> pqr_dot/1
  Demux/5 -> pqr_dot/2
  Demux/6 -> pqr_dot/3
  Bus Selector/2 -> Vrw_mag/2  "<V_rw_mag_eas>"
  Demux1/5 -> pqr/2
  Demux1/6 -> pqr/3
  Demux1/3 -> uvw/3
  Demux1/4 -> pqr/1
  Demux1/2 -> uvw/2
  Demux1/1 -> uvw/1
  Demux2/6 -> Radians to Degrees2/1
  Demux2/1 -> xyz/1
  Demux2/2 -> xyz/2
  Demux2/3 -> xyz/3
  Radians to Degrees2/1 -> phithetapsi/3
  Demux2/5 -> Radians to Degrees4/1
  Radians to Degrees4/1 -> phithetapsi/2
  Demux2/4 -> Radians to Degrees3/1
  Radians to Degrees3/1 -> phithetapsi/1

== system UNIFIER1/C7A_HARW/Subsystems ==
  X4 : Inport
  u1_in (rad) : Inport  Port=2
  u2 (actf) : Inport  Port=3
  u3 (actf) : Inport  Port=4
  sidestick_bus : Inport  Port=5
  X3 : Inport  Port=6
  X2 : Inport  Port=7
  Actuators : Subsystem
  DEP : Subsystem
  Gravity : Subsystem
  HTU : Subsystem
  LandingGears : Subsystem
  Scope : Scope
  Scopes : Subsystem
  Sum : Sum  Inputs=++++
  Sum1 : Sum  Inputs=+++
  Sum2 : Sum  Inputs=|++
  DEP_J : Outport
  u1_out (rad) : Outport  Port=2
  F : Outport  Port=3
  M : Outport  Port=4
  wires:
  X2/1 -> LandingGears/1(X2), DEP/1(X2)
  X4/1 -> DEP/2(X4), Gravity/1(X4), HTU/2(X4)
  DEP/1(DEP_J) -> DEP_J/1
  Sum/1 -> F/1
  Gravity/1(F) -> Sum/2
  HTU/1(F (N)) -> Sum/3
  Sum1/1 -> M/1
  HTU/2(M (Nm)) -> Sum1/2
  DEP/2(F) -> Sum/1
  DEP/3(M) -> Sum1/1
  u1_in (rad)/1 -> Scopes/2(cmd), Actuators/1(u1)
  Actuators/1(u1_actual) -> Scopes/1(actual), u1_out (rad)/1
  u3 (actf)/1 -> HTU/1(u3 (actf))
  DEP/4(P (kW)) -> Sum2/1
  HTU/3(P (kW)) -> Sum2/2
  u2 (actf)/1 -> DEP/3(u2 (actf))
  LandingGears/1(F) -> Sum/4
  LandingGears/2(M) -> Sum1/3
  X3/1 -> LandingGears/2(X3)
  sidestick_bus/1 -> LandingGears/3(sidestick_bus)
  Sum2/1 -> Scope/1

== system UNIFIER1/FCC/Airspeed Control ==
  note: swtich criteria:
      | 0 = real input
      | 1 = test (step) input
  Va : Inport
  Xe : Inport  Port=2
  1-D Lookup Table : Lookup_n-D  NumberOfTableDimensions=1  BreakpointsForDimension1=solution.X(:,1)  Table=Va  InternalRulePriority=Speed  RndMeth=Simplest
  Bus Creator : BusCreator  Inputs=2
  Constant : Constant  Value=0
  PID_Va : slpidlib/PID Controller  Controller=PID  Form=Parallel  TimeDomain=Continuous-time  UseExternalTs=off  SampleTime=-1  IntegratorMethod=Forward Euler  FilterMethod=Forward Euler  ControllerParametersSource=internal  P=0.85  I=0.038  UseKiTs=off  D=0  N=100  UseFilter=on  TunerSelectOption=Transfer Function Based (PID Tuner App)  InitialConditionSource=internal  InitialConditionForIntegrator=0  InitialConditionForFilter=0  DifferentiatorICPrevScaledInput=0  ExternalReset=none  TrackingMode=off  Kt=1  LimitOutput=off  SatLimitsSource=internal  UpperSaturationLimit=inf  LowerSaturationLimit=-inf  LinearizeAsGain=on  AntiWindupMode=none  Kb=1  LimitIntegrator=off  UpperIntegratorSaturationLimit=inf  LowerIntegratorSaturationLimit=-inf  POutMin=[]  POutMax=[]  IOutMin=[]  IOutMax=[]  DOutMin=[]  DOutMax=[]  NOutMin=[]  NOutMax=[]  SumOutMin=[]  SumOutMax=[]  SaturationOutMin=[]  SaturationOutMax=[]  PParamMin=[]  PParamMax=[]  IParamMin=[]  IParamMax=[]  DParamMin=[]  DParamMax=[]  NParamMin=[]  NParamMax=[]  KbParamMin=[]  KbParamMax=[]  KtParamMin=[]  KtParamMax=[]  KbOutMin=[]  KbOutMax=[]  KtOutMin=[]  KtOutMax=[]  IntegratorOutMin=[]  IntegratorOutMax=[]  FilterOutMin=[]  FilterOutMax=[]  SumI1OutMin=[]  SumI1OutMax=[]  SumI2OutMin=[]  SumI2OutMax=[]  SumI3OutMin=[]  SumI3OutMax=[]  SumI4OutMin=[]  SumI4OutMax=[]  SumDOutMin=[]  SumDOutMax=[]  DifferentiatorOutMin=[]  DifferentiatorOutMax=[]  FilterDiffOutCoefMin=[]  FilterDiffOutCoefMax=[]  ReciprocalOutMin=[]  ReciprocalOutMax=[]  SumDenOutMin=[]  SumDenOutMax=[]  SumNumOutMin=[]  SumNumOutMax=[]  DivideOutMin=[]  DivideOutMax=[]  UdiffTsProdOutMin=[]  UdiffTsProdOutMax=[]  NTsProdOutMin=[]  NTsProdOutMax=[]  UintegralTsProdOutMin=[]  UintegralTsProdOutMax=[]  UngainTsProdOutMin=[]  UngainTsProdOutMax=[]  ClampingZeroOutDataTypeStr=Inherit: Inherit via back propagation  ClampingZeroOutMin=[]  ClampingZeroOutMax=[]  FilterDenConstantOutDataTypeStr=Inherit: Inherit via back propagation  FilterDenConstantOutMin=[]  FilterDenConstantOutMax=[]  PCopyOutDataTypeStr=Inherit: Inherit via back propagation  PCopyOutMin=[]  PCopyOutMax=[]  NCopyOutDataTypeStr=Inherit: Inherit via back propagation  NCopyOutMin=[]  NCopyOutMax=[]  IntegratorContinuousStateAttributes=''  IntegratorStateMustResolveToSignalObject=off  IntegratorRTWStateStorageClass=Auto  FilterContinuousStateAttributes=''  FilterStateMustResolveToSignalObject=off  FilterRTWStateStorageClass=Auto  ParallelPVariant=InternalParameters  IdealPVariant=Disabled  IVariant=InternalParameters  DVariant=InternalParameters  IntegratorVariant=Continuous  SatVariant=Disabled  AWVariant=Passthrough  PCopyVariant=Disabled  TRVariant=Disabled  FdbkBlocksVariant=Forward  IdealPFdbkVariant=Disabled  SatFdbkVariant=Disabled  DerivativeFilterVariant=ContFilter  NVariant=InternalParameters  NCopyVariant=Disabled  FilterICVariant=InternalICsFilter  IntegratorICVariant=InternalICs  ExternalResetVariant=Disabled  TRSumVariant=Passthrough  SumFdbkVariant=Disabled  SumVariant=Sum_PID  TsampFilterVariant=InternalTs  TsampNgainVariant=Passthrough  TsampIntegralVariant=Disabled_SignalSpec  ExternalSaturationOutDataTypeStr=Inherit: Same as second input
  Sum : Sum  Inputs=|+-
  Switch : Switch  Criteria=u2 > Threshold  SaturateOnIntegerOverflow=off  InputSameDT=off
  Va_step : Step  Time=5  Before=72.74  After=72.74  SampleTime=0
  thr : Outport
  scopeout : Outport  Port=2
  wires:
  Va/1 -> Sum/2
  Sum/1 -> PID_Va/1
  PID_Va/1 -> thr/1, Bus Creator/2  "thr_cmd"
  Xe/1 -> 1-D Lookup Table/1
  1-D Lookup Table/1 -> Switch/3
  Switch/1 -> Bus Creator/1, Sum/1  "Va_ref"
  Bus Creator/1 -> scopeout/1
  Va_step/1 -> Switch/1
  Constant/1 -> Switch/2
